simulink model "Simulacion_sistema_con_controlador_LQR"  (R2021b)
settings: Solver=VariableStepAuto  StartTime=0.0  StopTime=5  FixedStep=0.01  RelTol=1e-3
model workspace (MATLAB code in the model file):
  | mCart = 1;
  | mPend = 1;
  | g = 9.81;
  | L = 0.5;
  | theta0 = 180;
  | Kd = 10;
undefined symbols (not defined in the file): A, B, b4, b5, b6, b7, b8, b9, C, K_LQR, Ke
settings Model: Creator=The MathWorks, Inc.  LastModifiedBy=Antonio
settings SolverCC: AlgebraicLoopSolver=TrustRegion
settings DataIOCC: TimeSaveName=T  SignalLoggingName=LoggedSigs
settings DebuggingCC: SFMachineParentedDataDiag=warning  ArithmeticOperatorsInVariantConditions=warning
settings SFSimCC: CustomCodeUndefinedFunction=UseInterfaceOnly
settings RTWCC: DLArmComputeVersion=20.02.1

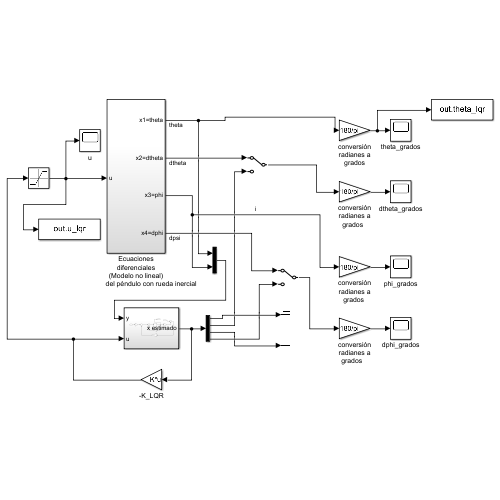
[thumbnail: Simulink's stored preview of the top-level diagram]
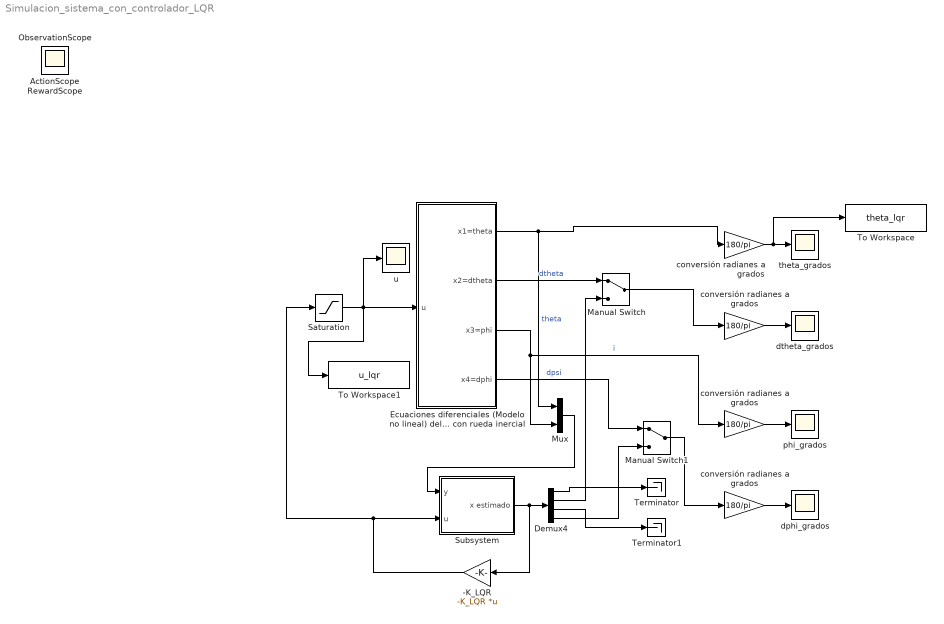
== system Simulacion_sistema_con_controlador_LQR ==
  -K_LQR : Gain  Gain=-K_LQR  Multiplication=Matrix(K*u)
  Demux4 : Demux
  Ecuaciones diferenciales (Modelo no lineal) del péndulo con rueda inercial : Subsystem
  Manual Switch : ManualSwitch
  Manual Switch1 : ManualSwitch
  Mux : Mux  Inputs=2
  Saturation : Saturate  UpperLimit=12  LowerLimit=-12
  Subsystem : Subsystem
  Terminator : Terminator
  Terminator1 : Terminator
  To Workspace : ToWorkspace  VariableName=theta_lqr  SampleTime=0.01
      settings: Save2DSignal=2-D array (concatenate along first dimension)
  To Workspace1 : ToWorkspace  VariableName=u_lqr  SampleTime=0.01
      settings: Save2DSignal=2-D array (concatenate along first dimension)
  conversión radianes a grados : Gain  Gain=180/pi
  "conversión radianes a grados " : Gain  Gain=180/pi
  "conversión radianes a grados  " : Gain  Gain=180/pi
  "conversión radianes a grados   " : Gain  Gain=180/pi
  dphi_grados : Scope
  dtheta_grados : Scope
  phi_grados : Scope
  theta_grados : Scope
  u : Scope
  ActionScope : Scope
  ObservationScope : Scope
  RewardScope : Scope
  wires:
  Ecuaciones diferenciales (Modelo no lineal) del péndulo con rueda inercial/4(x4=dphi) -> Manual Switch1/1  "dpsi"
  Manual Switch/1 -> "conversión radianes a grados  "/1
  Demux4/3 -> Terminator1/1
  Demux4/4 -> Manual Switch1/2
  Subsystem/1(x estimado) -> -K_LQR/1, Demux4/1
  Manual Switch1/1 -> "conversión radianes a grados   "/1
  Demux4/1 -> Terminator/1
  Mux/1 -> Subsystem/1(y)
  Ecuaciones diferenciales (Modelo no lineal) del péndulo con rueda inercial/2(x2=dtheta) -> Manual Switch/1  "dtheta"
  "conversión radianes a grados   "/1 -> dphi_grados/1
  "conversión radianes a grados "/1 -> phi_grados/1
  conversión radianes a grados/1 -> To Workspace/1, theta_grados/1
  "conversión radianes a grados  "/1 -> dtheta_grados/1
  Ecuaciones diferenciales (Modelo no lineal) del péndulo con rueda inercial/1(x1=theta) -> conversión radianes a grados/1, Mux/1  "theta"
  Ecuaciones diferenciales (Modelo no lineal) del péndulo con rueda inercial/3(x3=phi) -> "conversión radianes a grados "/1, Mux/2  "i"
  Demux4/2 -> Manual Switch/2
  -K_LQR/1 -> Saturation/1, Subsystem/2(u)
  Saturation/1 -> u/1, To Workspace1/1, Ecuaciones diferenciales (Modelo no lineal) del péndulo con rueda inercial/1(u)

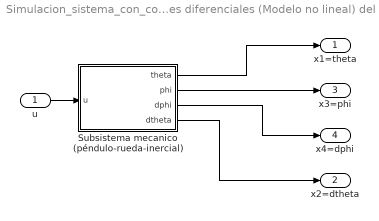
== system Simulacion_sistema_con_controlador_LQR/Ecuaciones diferenciales (Modelo no lineal) del péndulo con rueda inercial ==
  u : Inport
  Subsistema mecanico (péndulo-rueda-inercial) : Subsystem
  x1=theta : Outport
  x2=dtheta : Outport  Port=2
  x3=phi : Outport  Port=3
  x4=dphi : Outport  Port=4
  wires:
  Subsistema mecanico (péndulo-rueda-inercial)/4(dtheta) -> x2=dtheta/1
  u/1 -> Subsistema mecanico (péndulo-rueda-inercial)/1(u)
  Subsistema mecanico (péndulo-rueda-inercial)/2(phi) -> x3=phi/1
  Subsistema mecanico (péndulo-rueda-inercial)/3(dphi) -> x4=dphi/1
  Subsistema mecanico (péndulo-rueda-inercial)/1(theta) -> x1=theta/1

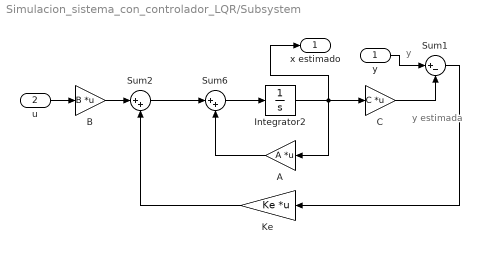
== system Simulacion_sistema_con_controlador_LQR/Subsystem ==
  note: y
  note: y estimada
  y : Inport
  u : Inport  Port=2
  A : Gain  Gain=A  Multiplication=Matrix(K*u)
  B : Gain  Gain=B  Multiplication=Matrix(K*u)
  C : Gain  Gain=C  Multiplication=Matrix(K*u)
  Integrator2 : Integrator
  Ke : Gain  Gain=Ke  Multiplication=Matrix(K*u)
  Sum1 : Sum  Inputs=|+-
  Sum2 : Sum  Inputs=|++
  Sum6 : Sum  Inputs=|++
  x estimado : Outport
  wires:
  C/1 -> Sum1/2
  Integrator2/1 -> x estimado/1, A/1, C/1
  Sum2/1 -> Sum6/1
  Ke/1 -> Sum2/2
  B/1 -> Sum2/1
  Sum6/1 -> Integrator2/1
  Sum1/1 -> Ke/1
  A/1 -> Sum6/2
  y/1 -> Sum1/1
  u/1 -> B/1

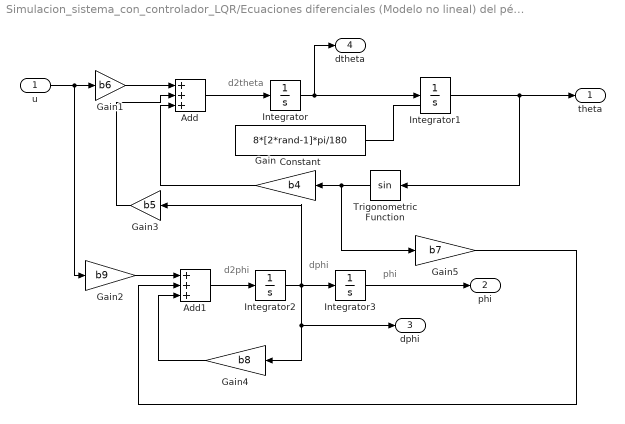
== system Simulacion_sistema_con_controlador_LQR/Ecuaciones diferenciales (Modelo no lineal) del péndulo con rueda inercial/Subsistema mecanico (péndulo-rueda-inercial) ==
  note: d2theta
  note: phi
  note: dphi
  note: d2phi
  u : Inport
  Add : Sum  Inputs=+++
  Add1 : Sum  Inputs=+++
  Constant : Constant  Value=8*[2*rand-1]*pi/180
  Gain : Gain  Gain=b4
  Gain1 : Gain  Gain=b6
  Gain2 : Gain  Gain=b9
  Gain3 : Gain  Gain=b5
  Gain4 : Gain  Gain=b8
  Gain5 : Gain  Gain=b7
  Integrator : Integrator
  Integrator1 : Integrator  InitialCondition=6*pi/180
  Integrator2 : Integrator
  Integrator3 : Integrator
  Trigonometric Function : Trigonometry
  theta : Outport
  phi : Outport  Port=2
  dphi : Outport  Port=3
  dtheta : Outport  Port=4
  wires:
  Add/1 -> Integrator/1
  Gain2/1 -> Add1/1
  Gain1/1 -> Add/1
  Add1/1 -> Integrator2/1
  Integrator1/1 -> Trigonometric Function/1, theta/1
  Integrator2/1 -> Gain3/1, dphi/1, Gain4/1, Integrator3/1
  u/1 -> Gain2/1, Gain1/1
  Trigonometric Function/1 -> Gain/1, Gain5/1
  Integrator3/1 -> phi/1
  Integrator/1 -> dtheta/1, Integrator1/1
  Gain/1 -> Add/3
  Gain3/1 -> Add/2
  Gain4/1 -> Add1/3
  Gain5/1 -> Add1/2
  Constant/1 -> ?
